simulink model "Libouga_Mbounja_SimulinkModelMatlab"  (R2018a)
settings: Solver=VariableStepAuto  StartTime=0.0  StopTime=50  MaxStep=1e-4  RelTol=1e-4
settings Model: Creator=root  LastModifiedBy=root

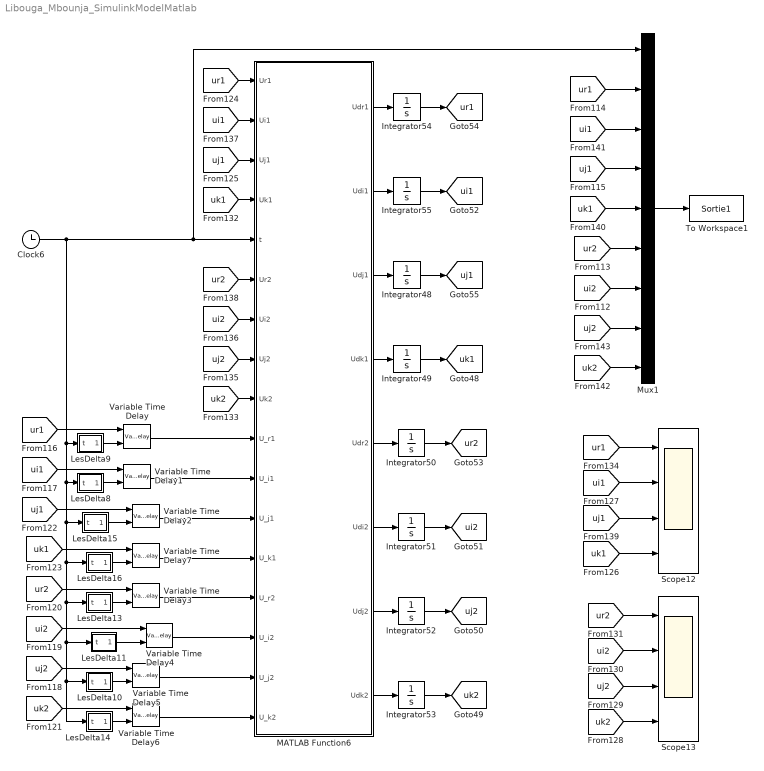
== system Libouga_Mbounja_SimulinkModelMatlab ==
  Clock6 : Clock
  Integrator{48..55} (8 alike) : Integrator
  LesDelta10 : MATLAB Function  TreatAsAtomicUnit=on
  LesDelta11 : MATLAB Function  TreatAsAtomicUnit=on
  LesDelta13 : MATLAB Function  TreatAsAtomicUnit=on
  LesDelta14 : MATLAB Function  TreatAsAtomicUnit=on
  LesDelta15 : MATLAB Function  TreatAsAtomicUnit=on
  LesDelta16 : MATLAB Function  TreatAsAtomicUnit=on
  LesDelta8 : MATLAB Function  TreatAsAtomicUnit=on
  LesDelta9 : MATLAB Function  TreatAsAtomicUnit=on
  MATLAB Function6 : MATLAB Function  TreatAsAtomicUnit=on
  Mux1 : Mux  Inputs=9
  Scope12 : Scope  NumInputPorts=4
  Scope13 : Scope  NumInputPorts=4
  To Workspace1 : ToWorkspace  VariableName=Sortie1  SampleTime=-1
  Variable Time Delay{,1..7} (8 alike) : VariableTransportDelay  MaximumDelay=10
  tag scope: ui1=global, ui2=global, uj1=global, uj2=global, uk1=global, uk2=global, ur1=global, ur2=global
  wires:
  [ur1] -> Mux1/2
  [uj2] -> Mux1/8
  [uj1] -> MATLAB Function6/3(Uj1)
  MATLAB Function6/8(Udk2) -> Integrator53/1
  Variable Time Delay/1 -> MATLAB Function6/10(U_r1)
  MATLAB Function6/6(Udi2) -> Integrator51/1
  [ur2] -> MATLAB Function6/6(Ur2)
  Variable Time Delay5/1 -> MATLAB Function6/16(U_j2)
  [ui2] -> Mux1/7
  MATLAB Function6/4(Udk1) -> Integrator49/1
  [ui1] -> Mux1/3
  Integrator50/1 -> [ur2]
  [uk2] -> Variable Time Delay6/1
  [ui1] -> MATLAB Function6/2(Ui1)
  MATLAB Function6/5(Udr2) -> Integrator50/1
  [uj2] -> MATLAB Function6/8(Uj2)
  Variable Time Delay4/1 -> MATLAB Function6/15(U_i2)
  Integrator48/1 -> [uj1]
  [ui2] -> Scope13/2
  [uk1] -> Mux1/5
  [uj1] -> Scope12/3
  [uk2] -> MATLAB Function6/9(Uk2)
  LesDelta16/1(y) -> Variable Time Delay7/2
  Integrator55/1 -> [ui1]
  LesDelta8/1(y) -> Variable Time Delay1/2
  [ur1] -> Scope12/1
  [uj2] -> Scope13/3
  [ui2] -> MATLAB Function6/7(Ui2)
  LesDelta14/1(y) -> Variable Time Delay6/2
  [ui2] -> Variable Time Delay4/1
  Variable Time Delay2/1 -> MATLAB Function6/12(U_j1)
  [uj2] -> Variable Time Delay5/1
  [ur2] -> Scope13/1
  [uk1] -> Variable Time Delay7/1
  MATLAB Function6/3(Udj1) -> Integrator48/1
  MATLAB Function6/1(Udr1) -> Integrator54/1
  MATLAB Function6/2(Udi1) -> Integrator55/1
  [uk2] -> Scope13/4
  [uj1] -> Mux1/4
  Variable Time Delay6/1 -> MATLAB Function6/17(U_k2)
  [uk2] -> Mux1/9
  LesDelta15/1(y) -> Variable Time Delay2/2
  Mux1/1 -> To Workspace1/1
  Integrator53/1 -> [uk2]
  [ui1] -> Scope12/2
  Integrator52/1 -> [uj2]
  [ur2] -> Mux1/6
  Variable Time Delay3/1 -> MATLAB Function6/14(U_r2)
  [uk1] -> MATLAB Function6/4(Uk1)
  Variable Time Delay1/1 -> MATLAB Function6/11(U_i1)
  LesDelta10/1(y) -> Variable Time Delay5/2
  [uk1] -> Scope12/4
  Integrator54/1 -> [ur1]
  Variable Time Delay7/1 -> MATLAB Function6/13(U_k1)
  [ur1] -> Variable Time Delay/1
  Integrator51/1 -> [ui2]
  LesDelta9/1(y) -> Variable Time Delay/2
  LesDelta11/1(y) -> Variable Time Delay4/2
  Clock6/1 -> LesDelta14/1(t), LesDelta10/1(t), LesDelta11/1(t), LesDelta13/1(t), LesDelta16/1(t), LesDelta15/1(t), LesDelta8/1(t), LesDelta9/1(t), Mux1/1, MATLAB Function6/5(t)
  [ur1] -> MATLAB Function6/1(Ur1)
  LesDelta13/1(y) -> Variable Time Delay3/2
  [ur2] -> Variable Time Delay3/1
  MATLAB Function6/7(Udj2) -> Integrator52/1
  [uj1] -> Variable Time Delay2/1
  [ui1] -> Variable Time Delay1/1
  Integrator49/1 -> [uk1]

== matlab function Libouga_Mbounja_SimulinkModelMatlab/LesDelta10 ==
  data: t input; y output
function y = fcn(t)

y= 0.2.*(abs(cos(sin(10*pi*t))));

== matlab function Libouga_Mbounja_SimulinkModelMatlab/LesDelta11 ==
  data: t input; y output
function y = fcn(t)

y= 0.2.*(abs(cos(sin(10*pi*t))));

== matlab function Libouga_Mbounja_SimulinkModelMatlab/LesDelta13 ==
  data: t input; y output
function y = fcn(t)

y= 0.2.*(abs(cos(sin(10*pi*t))));

== matlab function Libouga_Mbounja_SimulinkModelMatlab/LesDelta14 ==
  data: t input; y output
function y = fcn(t)

y= 0.2.*(abs(cos(sin(10*pi*t))));

== matlab function Libouga_Mbounja_SimulinkModelMatlab/LesDelta15 ==
  data: t input; y output
function y = fcn(t)

y= 0.2.*(abs(cos(sin(10*pi*t))));

== matlab function Libouga_Mbounja_SimulinkModelMatlab/LesDelta16 ==
  data: t input; y output
function y = fcn(t)

y= 0.2.*(abs(cos(sin(10*pi*t))));

== matlab function Libouga_Mbounja_SimulinkModelMatlab/LesDelta8 ==
  data: t input; y output
function y = fcn(t)

y= 0.2.*(abs(cos(sin(10*pi*t))));

== matlab function Libouga_Mbounja_SimulinkModelMatlab/LesDelta9 ==
  data: t input; y output
function y = fcn(t)

y= 0.2.*(abs(cos(sin(10*pi*t))));

== matlab function Libouga_Mbounja_SimulinkModelMatlab/MATLAB Function6 ==
  data: Ur1 input; Udr1 output; Ui1 input; Uj1 input; Uk1 input; t input; Ur2 input; Ui2 input; Uj2 input; Uk2 input; Udi1 output; Udj1 output; Udk1 output; Udr2 output; Udi2 output; Udj2 output; Udk2 output; U_r1 input; U_i1 input; U_j1 input; U_k1 input; U_r2 input; U_i2 input; U_j2 input; U_k2 input

function [Udr1,Udi1,Udj1,Udk1, Udr2,Udi2,Udj2,Udk2 ]= fcn(Ur1,Ui1,Uj1,Uk1,t, Ur2,Ui2,Uj2,Uk2, U_r1,U_i1,U_j1,U_k1, U_r2,U_i2,U_j2,U_k2)

% LES FONCTIONS QUATERNIONIQUES UTILISEES
% Gamma1 et Gamma2 
Gamma1 = 5+cos(sin(10*pi.*t))+ Phi(t);     Gamma2 =4+ cos(sin(10*pi.*t))+ Phi(t);
% Les fonctions Alpha
Alpha11 = quaternion(0.3*sin(10*pi.*t), 0.4*sin(10*pi.*t), 0.3*sin(10*pi.*t), 0.2*cos(10*pi.*t));
Alpha12 = quaternion(0.1*cos(10*pi.*t), 0.3*sin(10*pi.*t), 0.2*sin(10*pi.*t), 0.1*sin(10*pi.*t));
Alpha21 = quaternion(0.2*sin(10*pi.*t), 0.1*cos(10*pi.*t), 0.3*sin(10*pi.*t), 0.2*sin(10*pi.*t));
Alpha22 = quaternion(0.3*cos(10*pi.*t), 0.2*sin(10*pi.*t), 0.1*cos(10*pi.*t), 0.3*cos(10*pi.*t));
% Les fonction composees h(u(t))
h1U1=quaternion((1/8)*(cos(Ur1 + Uj1)).^2 ,(1/2)*abs(Ui1 + Uk1), (1/4)*cos(Uj1), (1/4).*(abs(Uk1+2)+abs(Uk1)-2));
h2U2=quaternion((1/8)*(cos(Ur2 + Uj2)).^2 ,(1/2)*abs(Ui2 + Uk2), (1/4)*cos(Uj2), (1/4).*(abs(Uk2+2)+abs(Uk2)-2));
% Les fonctions Beta
Beta11 = quaternion(0.1*cos(10*pi.*t)+ 0.1*Phi(t), 0.4*sin(10*pi.*t)+ 0.1*Phi(t), 0.1*sin(10*pi.*t)+ 0.1*Phi(t), 0.05*cos(10*pi.*t)+ 0.05*Phi(t));
Beta12 = quaternion(0.05*sin(10*pi.*t)+ 0.05*Phi(t), 0.2*cos(10*pi.*t)+ 0.1*Phi(t), 0.1*sin(10*pi.*t)+ 0.1*Phi(t), 0.1*cos(10*pi.*t)+ 0.1*Phi(t));
Beta21 = quaternion(0.05*cos(10*pi.*t)+ 0.05*Phi(t), 0.4*cos(10*pi.*t)+ 0.1*Phi(t), 0.1*sin(10*pi.*t)+ 0.1*Phi(t), 0.1*sin(10*pi.*t)+ 0.1*Phi(t));
Beta22 = quaternion(0.1*cos(10*pi.*t)+ 0.1*Phi(t), 0.2*cos(10*pi.*t)+ 0.1*Phi(t), 0.05*sin(10*pi.*t)+ 0.05*Phi(t), 0.1*cos(10*pi.*t)+ 0.1*Phi(t));
% Les fonctions Omega
Omega1 = quaternion(0.1*cos(10*pi.*t)+ 0.1*Phi(t), 0.1*sin(10*pi.*t)+ 0.1*Phi(t), 0.2*cos(10*pi.*t)+ 0.1*Phi(t), 0.05*cos(10*pi.*t)+ 0.05*Phi(t));
Omega2 = quaternion(0.3*sin(10*pi.*t)+ 0.1*Phi(t), 0.1*cos(10*pi.*t)+ 0.1*Phi(t), 0.1*cos(10*pi.*t)+ 0.1*Phi(t), 0.1*sin(10*pi.*t)+ 0.1*Phi(t));
% Les fonctions I
I1 = quaternion(0.1*sin(10*pi.*t)+ 0.1*Phi(t), 0.4*sin(10*pi.*t)+ 0.1*Phi(t), 0.1*cos(10*pi.*t)+ 0.1*Phi(t), 0.05*cos(10*pi.*t)+ 0.05*Phi(t));
I2 = quaternion(0.3*sin(10*pi.*t)+ 0.1*Phi(t), 0.1*cos(10*pi.*t)+ 0.1*Phi(t), 0.1*cos(10*pi.*t)+ 0.1*Phi(t), 0.1*sin(10*pi.*t)+ 0.1*Phi(t));
% Les fonctions T(t)
T11 = quaternion(0.05*sin(10*pi.*t)+ 0.05*Phi(t), 0.1*sin(10*pi.*t)+ 0.1*Phi(t), 0.6*cos(10*pi.*t)+ 0.1*Phi(t), 0.1*cos(10*pi.*t)+ 0.1*Phi(t));
T12 = quaternion(0.1*sin(10*pi.*t)+ 0.1*Phi(t), 0.4*cos(10*pi.*t)+ 0.1*Phi(t), 0.6*cos(10*pi.*t)+ 0.1*Phi(t), 0.05*cos(10*pi.*t)+ 0.05*Phi(t));
T21 = quaternion(0.1*sin(10*pi.*t)+ 0.1*Phi(t), 0.3*cos(10*pi.*t)+ 0.1*Phi(t), 0.1*cos(10*pi.*t)+ 0.1*Phi(t), 0.05*cos(10*pi.*t)+ 0.05*Phi(t));
T22 = quaternion(0.05*sin(10*pi.*t)+ 0.05*Phi(t), 0.3*cos(10*pi.*t)+ 0.1*Phi(t), 0.2*sin(10*pi.*t)+ 0.1*Phi(t), 0.05*cos(10*pi.*t)+ 0.05*Phi(t));
% Les fonctions H(t)
H11 = quaternion(0.1*sin(10*pi.*t)+ 0.1*Phi(t), 0.3*cos(10*pi.*t)+ 0.1*Phi(t), 0.4*sin(10*pi.*t)+ 0.1*Phi(t), 0.1*sin(10*pi.*t)+ 0.1*Phi(t));
H12 = quaternion(0.1*cos(10*pi.*t)+ 0.1*Phi(t), 0.05*cos(10*pi.*t)+ 0.05*Phi(t), 0.1*cos(10*pi.*t)+ 0.1*Phi(t), 0.05*cos(10*pi.*t)+ 0.05*Phi(t));
H21 = quaternion(0.2*sin(10*pi.*t)+ 0.1*Phi(t), 0.3*cos(10*pi.*t)+ 0.1*Phi(t), 0.2*sin(10*pi.*t)+ 0.1*Phi(t), 0.05*cos(10*pi.*t)+ 0.05*Phi(t));
H22 = quaternion(0.3*sin(10*pi.*t)+ 0.1*Phi(t), 0.1*sin(10*pi.*t)+ 0.1*Phi(t), 0.2*sin(10*pi.*t)+ 0.1*Phi(t), 0.05*cos(10*pi.*t)+ 0.05*Phi(t));
% Les fonctions a(t)
a11 = quaternion(0.5*cos(10*pi.*t), 0.1*cos(10*pi.*t), 0.3*sin(10*pi.*t), 0.4*cos(10*pi.*t));
a12 = quaternion(0.3*cos(10*pi.*t), 0.4*cos(10*pi.*t), 0.1*sin(10*pi.*t), 0.3*cos(10*pi.*t));
a21 = quaternion(0.3*sin(10*pi.*t), 0.4*sin(10*pi.*t), 0.1*sin(10*pi.*t), 0.1*cos(10*pi.*t));
a22 = quaternion(0.2*cos(10*pi.*t), 0.4*sin(10*pi.*t), 0.1*sin(10*pi.*t), 0.1*cos(10*pi.*t));
% Les fonctions b(t)
b11 = quaternion(0.3*sin(10*pi.*t), 0.6*cos(10*pi.*t), 0.1*sin(10*pi.*t), 0.2*cos(10*pi.*t));
b12 = quaternion(0.5*cos(10*pi.*t), 0.6*cos(10*pi.*t), 0.2*cos(10*pi.*t), 0.2*cos(10*pi.*t));
b21 = quaternion(0.2*cos(10*pi.*t), 0.4*sin(10*pi.*t), 0.2*cos(10*pi.*t), 0.2*sin(10*pi.*t));
b22 = quaternion(0.6*cos(10*pi.*t), 0.1*sin(10*pi.*t), 0.7*cos(10*pi.*t), 0.2*cos(10*pi.*t));
% Les fonction composees delay p(u(t-delta)) et q(u(t-delta))
P1U1=quaternion((1/8)*(sin(U_r1 + U_j1)).^2 ,(1/2)*abs(U_i1 + U_k1), (1/4)*sin(U_j1), (1/8).*(abs(U_k1+0.5)+abs(U_k1)-0.5));
P2U2=quaternion((1/8)*(sin(U_r2 + U_j2)).^2 ,(1/2)*abs(U_i2 + U_k2), (1/4)*sin(U_j2), (1/8).*(abs(U_k2+0.5)+abs(U_k2)-0.5));
Q1U1=quaternion((1/2)*(tan(U_j1)) ,(sin(U_r1 + U_i1)).^2, (1/2)*abs(U_j1), cos(10*pi.*U_k1));
Q2U2=quaternion((1/2)*(tan(U_j2)) ,(sin(U_r2 + U_i2)).^2, (1/2)*abs(U_j2), cos(10*pi.*U_k2));
% des produits
AP1= a11*P1U1; AP2= a12*P2U2; AP3= a21*P1U1; AP4= a22*P2U2; 
AP= ETQuart(AP1,AP2); A_P= ETQuart(AP3,AP4);

BQ1= b11*Q1U1; BQ2= b12*Q2U2; BQ3= b21*Q1U1; BQ4= b22*Q2U2; 
BQ= ETQuart(BQ1,BQ2); B_Q= ETQuart(BQ3,BQ4);

TO1= T11*Omega1; TO2= T12*Omega2; TO3= T21*Omega1; TO4= T22*Omega2; 
TO= ETQuart(TO1,TO2); T_O= ETQuart(TO3,TO4);

HO1= H11*Omega1; HO2= H12*Omega2; HO3= H21*Omega1; HO4= H22*Omega2; 
HO= OUQuart(HO1,HO2); H_O= OUQuart(HO3,HO4);


% CONSTRUCTION DES QUATERNIONS U1 et U2
Uq1 = quaternion(Ur1,Ui1,Uj1,Uk1) ;  Uq2 = quaternion(Ur2,Ui2,Uj2,Uk2);


% EQUATIONS DIFFERENTIELLES
Udq1 = (-Gamma1 .* Uq1) + (Alpha11 * h1U1) + (Alpha12 * h2U2) + (Beta11 * Omega1) + (Beta12 * Omega2) + I1 + AP + BQ + TO + HO ; 
Udq2 = (-Gamma2 .* Uq2) + (Alpha21 * h1U1) + (Alpha22 * h2U2) + (Beta21 * Omega1) + (Beta22 * Omega2) + I2 + A_P + B_Q + T_O + H_O; 


% EXTRACTION DES PARTIES DES QUATERNIONS
[Udr1,Udi1,Udj1,Udk1] = parts(Udq1);   [Udr2,Udi2,Udj2,Udk2] = parts(Udq2);

end

function [P]=Phi(a)
if a>0
    P=0;
else
    P=exp(-a);
end
end



function [C] = ETQuart(A,B)   
[R1,I_1,J1,K1] = parts(A);   [R2,I_2,J2,K2] = parts(B);
R3 = (R1 & R2) - (I_1 & I_2) - (J1 & J2) - (K1 & K2);
I3 = (R1 & I_2) + (I_1 & R2) + (J1 & K2) - (K1 & J2);
J3 = (R1 & J2) + (J1 & R2) +  (K1 & I_2) - (I_1 & K2);
K3 = (R1 & K2) + (K1 & R2) + (I_1 & J2) - (J1 & I_2);
C = quaternion(R3,I3,J3,K3) ;
end

function [C] = OUQuart(A,B)   
[R1,I_1,J1,K1] = parts(A);   [R2,I_2,J2,K2] = parts(B);
R3 = (R1 | R2) - (I_1 | I_2) - (J1 | J2) - (K1 | K2);
I3 = (R1 | I_2) + (I_1 | R2) + (J1 | K2) - (K1 | J2);
J3 = (R1 | J2) + (J1 | R2) +  (K1 | I_2) - (I_1 | K2);
K3 = (R1 | K2) + (K1 | R2) + (I_1 | J2) - (J1 | I_2);
C = quaternion(R3,I3,J3,K3) ;
end
